simulink model "fixed_wing_sim"  (Simulink 8.7)
settings: Solver=ode4  StartTime=0.0  StopTime=T_sim  FixedStep=ts_sim  MaxStep=10e-3  RelTol=1e-3
InitFcn:
  | % Run the initialization script
  | clear all
  | aerosonde_uav_conf_model
StopFcn:
  | %show_result
  | print_results
values from neighbouring files (symbols this model uses):
  a = param(1)    [get_field.m]    (also in print_results.m = a*scale_fac/1e3; vector_field_parameters.m = 0.85)
  AilBnd = range_ail.*degrees2rad    [aerosonde_uav_conf_model.m]
  aileron_limits = [-20*pi/180;20*pi/180]    [aerosonde_uav_conf_model.m]
  AlphaBnd = range_alpha.*degrees2rad    [aerosonde_uav_conf_model.m]
  amp_theta = amp_theta*2    [vector_field_parameters.m]
  amp_theta_c = ((1/4)*[1 1 1]/6)*U_theta*tau_theta    [vector_field_parameters.m]
  amp_v_c = [1 1 1]*(tau_v*U_v)/6    [vector_field_parameters.m]
  amp_x = [5 5 5]    [vector_field_parameters.m]
  amp_y = [5 5 5]    [vector_field_parameters.m]
  amp_z = amp_z*2    [vector_field_parameters.m]
  amp_z_c = [1 1 1]*(tau_z*U_z)/6/2    [vector_field_parameters.m]
  b = param(2)    [get_field.m]    (also in print_results.m = b*scale_fac/1e3; vector_field_parameters.m = 0.08)
  BetaBnd = range_beta.*degrees2rad    [aerosonde_uav_conf_model.m]
  Bw = 2.8956    [aerosonde_uav_conf_model.m]
  c = param(3)    [get_field.m]    (also in vector_field_parameters.m = -0.13)
  CD_0 = 0.0434    [aerosonde_uav_conf_model.m]
  CD_ail = ones(length(AlphaBnd),1)*CD_aux_ail    [aerosonde_uav_conf_model.m]
  CD_alpha_beta = zeros(length(AlphaBnd),length(BetaBnd))    [aerosonde_uav_conf_model.m]
  CD_elev = ones(length(AlphaBnd),1)*CD_aux_elev    [aerosonde_uav_conf_model.m]
  CD_mind = 0.23    [aerosonde_uav_conf_model.m]
  CD_rud = ones(length(AlphaBnd),1)*CD_aux_rud    [aerosonde_uav_conf_model.m]
  CL_0 = 0.23    [aerosonde_uav_conf_model.m]
  Cl_ail = ones(length(AlphaBnd),1)*Cl_aux_ail    [aerosonde_uav_conf_model.m]
  CL_alpha_beta = CL_alpha*ones(1,length(BetaBnd))    [aerosonde_uav_conf_model.m]
  Cl_alpha_beta = ones(length(AlphaBnd),1)*Cl_beta    [aerosonde_uav_conf_model.m]
  CL_alphadot = 1.9724    [aerosonde_uav_conf_model.m]
  CL_elev = ones(length(AlphaBnd),1)*CL_aux_elev    [aerosonde_uav_conf_model.m]
  Cl_P = ones(length(AlphaBnd),1)*Cl_aux_P    [aerosonde_uav_conf_model.m]
  CL_Q = 7.9543*QBnd    [aerosonde_uav_conf_model.m]
  Cl_R = ones(length(AlphaBnd),1)*Cl_aux_R    [aerosonde_uav_conf_model.m]
  Cl_rud = ones(length(AlphaBnd),1)*Cl_aux_rud    [aerosonde_uav_conf_model.m]
  CLE_alphat = zeros(1,length(AlphaBnd))    [aerosonde_uav_conf_model.m]
  CLE_elev = 0    [aerosonde_uav_conf_model.m]
  Cm0 = 0.135    [aerosonde_uav_conf_model.m]
  Cm_alpha_beta = Cm_alpha*ones(1,length(BetaBnd))    [aerosonde_uav_conf_model.m]
  Cm_alphadot = -10.3796    [aerosonde_uav_conf_model.m]
  Cm_elev = ones(length(AlphaBnd),1)*Cm_aux_elev    [aerosonde_uav_conf_model.m]
  Cm_Q = -38.2067*QBnd    [aerosonde_uav_conf_model.m]
  Cn_ail = ones(length(AlphaBnd),1)*Cn_aux_ail    [aerosonde_uav_conf_model.m]
  Cn_alpha_beta = ones(length(AlphaBnd),1)*Cn_beta    [aerosonde_uav_conf_model.m]
  Cn_P = ones(length(AlphaBnd),1)*Cn_aux_P    [aerosonde_uav_conf_model.m]
  Cn_R = ones(length(AlphaBnd),1)*Cn_aux_R    [aerosonde_uav_conf_model.m]
  Cn_rud = ones(length(AlphaBnd),1)*Cn_aux_rud    [aerosonde_uav_conf_model.m]
  CT_save = CT_save.*10    [aerosonde_uav_conf_model.m]    (also in helice.mat = [0.115262 0.00375054783545 -0.00666475255621 -0.006665219028)
  curve = 1    [vector_field_parameters.m]
  Cw = 0.189941    [aerosonde_uav_conf_model.m]
  CY_ail = ones(length(AlphaBnd),1)*CY_aux_ail    [aerosonde_uav_conf_model.m]
  CY_alpha_beta = ones(length(AlphaBnd),1)*CY_beta    [aerosonde_uav_conf_model.m]
  CY_P = zeros(length(AlphaBnd),length(PBnd))    [aerosonde_uav_conf_model.m]
  CY_R = zeros(length(AlphaBnd),length(RBnd))    [aerosonde_uav_conf_model.m]
  CY_rud = ones(length(AlphaBnd),1)*CY_aux_rud    [aerosonde_uav_conf_model.m]
  d = param(4)    [get_field.m]    (also in vector_field_parameters.m = -0.04)
  D_hel = 0.15    [aerosonde_uav_conf_model.m]
  d_wash = 0    [aerosonde_uav_conf_model.m]
  delta_CD = 1    [aerosonde_uav_conf_model.m]
  delta_CL = 1    [aerosonde_uav_conf_model.m]
  delta_Cl = 1    [aerosonde_uav_conf_model.m]
  delta_Cm = 1    [aerosonde_uav_conf_model.m]
  delta_Cn = 1    [aerosonde_uav_conf_model.m]
  delta_CY = 1    [aerosonde_uav_conf_model.m]
  delta_FT = 1    [aerosonde_uav_conf_model.m]
  Delta_V_EH = [ 2 1.7365 1.2985 1.0890 1.0205]    [aerosonde_uav_conf_model.m]
  Delta_V_J = [ 0 0.4 0.7 1.4 2.1]    [aerosonde_uav_conf_model.m]
  elevator_limits = [-15*pi/180;15*pi/180]    [aerosonde_uav_conf_model.m]
  ElevBnd = range_elev.*degrees2rad    [aerosonde_uav_conf_model.m]
  F_T = 19    [aerosonde_uav_conf_model.m]
  f_theta = ([5 3 1]+rand(1,3))*0.05*2*pi/freq_divisor    [vector_field_parameters.m]
  f_theta_c = ([5 3 1]+rand(1,3))*0.05*2*pi/freq_divisor    [vector_field_parameters.m]
  f_v_c = ([4 2 0.5]+rand(1,3))*0.05*2*pi/freq_divisor    [vector_field_parameters.m]
  f_x = ([6 4 2]+rand(1,3))*0.05*2*pi/freq_divisor    [vector_field_parameters.m]
  f_y = ([6 4 2]+rand(1,3))*0.05*2*pi/freq_divisor    [vector_field_parameters.m]
  f_z = ([6 4 2]+rand(1,3))*0.05*2*pi/freq_divisor    [vector_field_parameters.m]
  f_z_c = ([4 2 0.5]+rand(1,3))*0.05*2*pi/freq_divisor    [vector_field_parameters.m]
  g1 = param(5)    [get_field.m]    (also in vector_field_parameters.m = 4)
  gain_G = param(6)    [get_field.m]    (also in vector_field_parameters.m = 2.5)
  gravity = 9.807    [aerosonde_uav_conf_model.m]
  H_0 = 200    [vector_field_parameters.m]
  Heq = 200    [aerosonde_uav_conf_model.m]    (also in vector_field_parameters.m)
  induced_drag = 1/(pi*AR*osw)    (= 0.0278403324809)    [aerosonde_uav_conf_model.m]
  isTrimming = 0    [aerosonde_uav_conf_model.m]
  J_save = J_save.*1.5    [aerosonde_uav_conf_model.m]    (also in helice.mat = [0 1.22229381539 1.27367709689 1.27367940534 1.27361400442 1)
  Jx = 0.7795    [aerosonde_uav_conf_model.m]
  Jxz = 0.1211    [aerosonde_uav_conf_model.m]
  Jy = 1.122    [aerosonde_uav_conf_model.m]
  Jz = 1.752    [aerosonde_uav_conf_model.m]
  KC_h = 0.28    [aerosonde_uav_conf_model.m]
  KC_phi = -1.18    [aerosonde_uav_conf_model.m]
  KC_psi = 0.03    [aerosonde_uav_conf_model.m]
  KC_r = -0.0073    [aerosonde_uav_conf_model.m]
  KC_theta = -1.1482    [aerosonde_uav_conf_model.m]
  KC_vt = 0.9948*1    (= 0.9948)    [aerosonde_uav_conf_model.m]
  KE = -0.1562    [aerosonde_uav_conf_model.m]
  Kp = 0.18    [vector_field_parameters.m]
  KR = 0.0130    (= 0.013)    [aerosonde_uav_conf_model.m]
  Ksad = param(3)    [get_field.m]    (also in print_results.m = Ksad*scale_fac/1e3; vector_field_parameters.m = 0)
  KT = 0.0792    [aerosonde_uav_conf_model.m]
  Kv = 1    [vector_field_parameters.m]
  LIM_CENTER = LIM_CENTER*scale_fac/1e3    [print_results.m]    (also in vector_field_parameters.m = 0.2)
  M = 8.5    [aerosonde_uav_conf_model.m]    (also in print_results.m = 0)
  motor_min = 0.1    [aerosonde_uav_conf_model.m]
  motor_rate = 1    [aerosonde_uav_conf_model.m]
  p_theta = rand(1,3)*2*pi    [vector_field_parameters.m]
  p_theta_c = rand(1,3)*2*pi    [vector_field_parameters.m]
  p_v_c = rand(1,3)*2*pi    [vector_field_parameters.m]
  p_x = rand(1,3)*2*pi    [vector_field_parameters.m]
  p_y = rand(1,3)*2*pi    [vector_field_parameters.m]
  p_z = rand(1,3)*2*pi    [vector_field_parameters.m]
  p_z_c = rand(1,3)*2*pi    [vector_field_parameters.m]
  PBnd = range_P.*degrees2rad    [aerosonde_uav_conf_model.m]
  perc_int_max = 0.8    [aerosonde_uav_conf_model.m]
  phi_max = 20*pi/180    (= 0.349065850399)    [aerosonde_uav_conf_model.m]
  phi_min = -20*pi/180    (= -0.349065850399)    [aerosonde_uav_conf_model.m]
  QBnd = range_Q.*degrees2rad    [aerosonde_uav_conf_model.m]
  r = sqrt(m)    [animation.m]    (also in print_results.m)
  r_aero_abc = r_aero_struct*[-1 0 0;0 1 0;0 0 -1]    [aerosonde_uav_conf_model.m]
  r_cg_abc = r_cg_struct*[-1 0 0;0 1 0;0 0 -1]    [aerosonde_uav_conf_model.m]
  r_motor_abc = r_motor_struct*[-1 0 0;0 1 0;0 0 -1]    [aerosonde_uav_conf_model.m]
  r_tail_abc = r_aero_struct*[-1 0 0;0 1 0;0 0 -1]    [aerosonde_uav_conf_model.m]
  RBnd = range_R.*degrees2rad    [aerosonde_uav_conf_model.m]
  rho = 0.1    [aerosonde_uav_conf_model.m]
  ... (+40 more)
undefined symbols (not defined in the file or in its folder): Earth, F, Light, MIL, WGS84
libraries: aerolibwind2 x2, aerolibtransform2 x2, aerolibfltsims x1, aerolibconvert2 x1, dspsigops x1
(part 3 of 3)

== system fixed_wing_sim/A/C + Low Level Control /UAV Internal Closed Loops/UAV model/Body-Axes 6DOF Equations/Moment Equations/Inverse Inertia Matrix ==
  Constant : Constant  Value=Jz
  Constant1 : Constant  Value=1/Jy
  Constant2 : Constant  Value=Jx
  Constant3 : Constant  Value=Jxz
  Constant4 : Constant  Value=0
  Constant5 : Constant  Value=Jx*Jz - Jxz^2
  Matrix Concatenation10 : Concatenate  NumInputs=3  Mode=Multidimensional array
  Matrix Concatenation11 : Concatenate  NumInputs=3  Mode=Multidimensional array  ConcatenateDimension=2
  Matrix Concatenation8 : Concatenate  NumInputs=3  Mode=Multidimensional array
  Matrix Concatenation9 : Concatenate  NumInputs=3  Mode=Multidimensional array
  Product : Product  Inputs=*/  SaturateOnIntegerOverflow=on  OutDataTypeStr=Inherit: Same as first input
  Product1 : Product  SaturateOnIntegerOverflow=on  OutDataTypeStr=Inherit: Same as first input
  inv J_b : Outport
  wires:
  Matrix Concatenation8/1 -> Matrix Concatenation11/1
  Matrix Concatenation9/1 -> Matrix Concatenation11/2
  Matrix Concatenation10/1 -> Matrix Concatenation11/3
  Constant/1 -> Matrix Concatenation8/1
  Constant4/1 -> Matrix Concatenation8/2, Matrix Concatenation9/1, Matrix Concatenation9/3, Matrix Concatenation10/2
  Constant3/1 -> Matrix Concatenation8/3, Matrix Concatenation10/1
  Constant2/1 -> Matrix Concatenation10/3
  Matrix Concatenation11/1 -> Product/1
  Product/1 -> inv J_b/1
  Constant5/1 -> Product/2, Product1/2
  Constant1/1 -> Product1/1
  Product1/1 -> Matrix Concatenation9/2

== system fixed_wing_sim/A/C + Low Level Control /UAV Internal Closed Loops/UAV model/Body-Axes 6DOF Equations/Moment Equations/Produto Vetorial1 ==
  V1 : Inport
  V2 : Inport  Port=2
  Mux : Mux  Inputs=2
  Mux1 : Mux  Inputs=3
  i : Fcn  Expr=u(2)*u(6)-u(3)*u(5)
  j : Fcn  Expr=-u(1)*u(6)+u(3)*u(4)
  k : Fcn  Expr=u(1)*u(5)-u(2)*u(4)
  V1 x V2 : Outport
  wires:
  V1/1 -> Mux/1
  V2/1 -> Mux/2
  Mux/1 -> i/1, j/1, k/1
  i/1 -> Mux1/1
  j/1 -> Mux1/2
  k/1 -> Mux1/3
  Mux1/1 -> V1 x V2/1

== system fixed_wing_sim/A/C + Low Level Control /UAV Internal Closed Loops/UAV model/Body-Axes 6DOF Equations/Moment Equations/Produto Vetorial2 ==
  V1 : Inport
  V2 : Inport  Port=2
  Mux : Mux  Inputs=2
  Mux1 : Mux  Inputs=3
  i : Fcn  Expr=u(2)*u(6)-u(3)*u(5)
  j : Fcn  Expr=-u(1)*u(6)+u(3)*u(4)
  k : Fcn  Expr=u(1)*u(5)-u(2)*u(4)
  V1 x V2 : Outport
  wires:
  V1/1 -> Mux/1
  V2/1 -> Mux/2
  Mux/1 -> i/1, j/1, k/1
  i/1 -> Mux1/1
  j/1 -> Mux1/2
  k/1 -> Mux1/3
  Mux1/1 -> V1 x V2/1

== system fixed_wing_sim/A/C + Low Level Control /UAV Internal Closed Loops/UAV model/Body-Axes 6DOF Equations/Moment Equations/Produto Vetorial3 ==
  V1 : Inport
  V2 : Inport  Port=2
  Mux : Mux  Inputs=2
  Mux1 : Mux  Inputs=3
  i : Fcn  Expr=u(2)*u(6)-u(3)*u(5)
  j : Fcn  Expr=-u(1)*u(6)+u(3)*u(4)
  k : Fcn  Expr=u(1)*u(5)-u(2)*u(4)
  V1 x V2 : Outport
  wires:
  V1/1 -> Mux/1
  V2/1 -> Mux/2
  Mux/1 -> i/1, j/1, k/1
  i/1 -> Mux1/1
  j/1 -> Mux1/2
  k/1 -> Mux1/3
  Mux1/1 -> V1 x V2/1

== system fixed_wing_sim/A/C + Low Level Control /UAV Internal Closed Loops/UAV model/Body-Axes 6DOF Equations/Moment Equations/Produto Vetorial4 ==
  V1 : Inport
  V2 : Inport  Port=2
  Mux : Mux  Inputs=2
  Mux1 : Mux  Inputs=3
  i : Fcn  Expr=u(2)*u(6)-u(3)*u(5)
  j : Fcn  Expr=-u(1)*u(6)+u(3)*u(4)
  k : Fcn  Expr=u(1)*u(5)-u(2)*u(4)
  V1 x V2 : Outport
  wires:
  V1/1 -> Mux/1
  V2/1 -> Mux/2
  Mux/1 -> i/1, j/1, k/1
  i/1 -> Mux1/1
  j/1 -> Mux1/2
  k/1 -> Mux1/3
  Mux1/1 -> V1 x V2/1

== system fixed_wing_sim/A/C + Low Level Control /UAV Internal Closed Loops/UAV model/Body-Axes 6DOF Equations/NED --> ABC/R_phi  ==
  note: 1       0      0
      | 0   cos   sin
      | 0  -sen  cos
  note: R_phi -->
  In1 : Inport
  Constant : Constant
  Constant1 : Constant  Value=0
  Gain : Gain  Gain=-1
  Matrix Concatenate : Concatenate  NumInputs=3  Mode=Multidimensional array
  Matrix Concatenate1 : Concatenate  NumInputs=3  Mode=Multidimensional array
  Matrix Concatenate2 : Concatenate  NumInputs=3  Mode=Multidimensional array
  Matrix Concatenate3 : Concatenate  NumInputs=3  Mode=Multidimensional array  ConcatenateDimension=2
  cos(phi) : Trigonometry  Operator=cos
  sin(phi) : Trigonometry
  Out1 : Outport
  wires:
  Constant/1 -> Matrix Concatenate/1
  Constant1/1 -> Matrix Concatenate/2, Matrix Concatenate/3, Matrix Concatenate1/1, Matrix Concatenate2/1
  cos(phi)/1 -> Matrix Concatenate1/2, Matrix Concatenate2/3
  sin(phi)/1 -> Gain/1, Matrix Concatenate2/2
  Gain/1 -> Matrix Concatenate1/3
  Matrix Concatenate/1 -> Matrix Concatenate3/1
  Matrix Concatenate1/1 -> Matrix Concatenate3/2
  Matrix Concatenate2/1 -> Matrix Concatenate3/3
  Matrix Concatenate3/1 -> Out1/1
  In1/1 -> cos(phi)/1, sin(phi)/1

== system fixed_wing_sim/A/C + Low Level Control /UAV Internal Closed Loops/UAV model/Body-Axes 6DOF Equations/NED --> ABC/R_psi ==
  note: cos  sin   0
      | -sin  cos  0
      | 0       0     1
  note: R_psi -->
  In1 : Inport
  Constant : Constant
  Constant1 : Constant  Value=0
  Gain : Gain  Gain=-1
  Matrix Concatenate : Concatenate  NumInputs=3  Mode=Multidimensional array
  Matrix Concatenate1 : Concatenate  NumInputs=3  Mode=Multidimensional array
  Matrix Concatenate2 : Concatenate  NumInputs=3  Mode=Multidimensional array
  Matrix Concatenate3 : Concatenate  NumInputs=3  Mode=Multidimensional array  ConcatenateDimension=2
  cos(phi) : Trigonometry  Operator=cos
  sin(phi) : Trigonometry
  Out1 : Outport
  wires:
  Matrix Concatenate/1 -> Matrix Concatenate3/1
  Matrix Concatenate1/1 -> Matrix Concatenate3/2
  Matrix Concatenate2/1 -> Matrix Concatenate3/3
  Matrix Concatenate3/1 -> Out1/1
  cos(phi)/1 -> Matrix Concatenate/1, Matrix Concatenate1/2
  Gain/1 -> Matrix Concatenate/2
  sin(phi)/1 -> Gain/1, Matrix Concatenate1/1
  Constant1/1 -> Matrix Concatenate/3, Matrix Concatenate1/3, Matrix Concatenate2/1, Matrix Concatenate2/2
  Constant/1 -> Matrix Concatenate2/3
  In1/1 -> cos(phi)/1, sin(phi)/1

== system fixed_wing_sim/A/C + Low Level Control /UAV Internal Closed Loops/UAV model/Body-Axes 6DOF Equations/NED --> ABC/R_theta ==
  note: cos  0 -sin
      | 0    1    0
      | sin   0  cos
  note: R_theta -->
  In1 : Inport
  Constant : Constant
  Constant1 : Constant  Value=0
  Gain : Gain  Gain=-1
  Matrix Concatenate : Concatenate  NumInputs=3  Mode=Multidimensional array
  Matrix Concatenate1 : Concatenate  NumInputs=3  Mode=Multidimensional array
  Matrix Concatenate2 : Concatenate  NumInputs=3  Mode=Multidimensional array
  Matrix Concatenate3 : Concatenate  NumInputs=3  Mode=Multidimensional array  ConcatenateDimension=2
  cos(phi) : Trigonometry  Operator=cos
  sin(phi) : Trigonometry
  Out1 : Outport
  wires:
  Matrix Concatenate/1 -> Matrix Concatenate3/1
  Matrix Concatenate1/1 -> Matrix Concatenate3/2
  Matrix Concatenate2/1 -> Matrix Concatenate3/3
  Matrix Concatenate3/1 -> Out1/1
  cos(phi)/1 -> Matrix Concatenate/1, Matrix Concatenate2/3
  Constant1/1 -> Matrix Concatenate/2, Matrix Concatenate1/1, Matrix Concatenate1/3, Matrix Concatenate2/2
  Constant/1 -> Matrix Concatenate1/2
  In1/1 -> cos(phi)/1, sin(phi)/1
  sin(phi)/1 -> Matrix Concatenate/3, Gain/1
  Gain/1 -> Matrix Concatenate2/1

== system fixed_wing_sim/A/C + Low Level Control /UAV Internal Closed Loops/UAV model/Body-Axes 6DOF Equations/Navigation Equations/ABC --> NED ==
  note: NED = (R_phi * R_theta * R_psi)^(T) * ABC
  attitude : Inport
  v_ABC : Inport  Port=2
  Bus Selector : BusSelector  OutputSignals=phi,theta,psi
  Math Function : Math  Operator=transpose  SaturateOnIntegerOverflow=on
  Product : Product  Multiplication=Matrix(*)  RndMeth=Zero
  Product1 : Product  Multiplication=Matrix(*)  RndMeth=Zero
  Product2 : Product  Multiplication=Matrix(*)  RndMeth=Zero
  "R_phi " : Subsystem
  R_psi : Subsystem
  R_theta : Subsystem
  NED : Outport
  wires:
  attitude/1 -> Bus Selector/1
  R_theta/1(Out1) -> Product/2
  Product/1 -> Product1/1
  "R_phi "/1(Out1) -> Product/1
  R_psi/1(Out1) -> Product1/2
  v_ABC/1 -> Product2/2
  Product2/1 -> NED/1
  Product1/1 -> Math Function/1
  Math Function/1 -> Product2/1
  Bus Selector/2 -> R_theta/1(In1)  "<theta>"
  Bus Selector/3 -> R_psi/1(In1)  "<psi>"
  Bus Selector/1 -> "R_phi "/1(In1)  "<phi>"

== system fixed_wing_sim/A/C + Low Level Control /UAV Internal Closed Loops/UAV model/Body-Axes 6DOF Equations/Force Equations/NED --> ABC/R_phi  ==
  note: 1       0      0
      | 0   cos   sin
      | 0  -sen  cos
  note: R_phi -->
  In1 : Inport
  Constant : Constant
  Constant1 : Constant  Value=0
  Gain : Gain  Gain=-1
  Matrix Concatenate : Concatenate  NumInputs=3  Mode=Multidimensional array
  Matrix Concatenate1 : Concatenate  NumInputs=3  Mode=Multidimensional array
  Matrix Concatenate2 : Concatenate  NumInputs=3  Mode=Multidimensional array
  Matrix Concatenate3 : Concatenate  NumInputs=3  Mode=Multidimensional array  ConcatenateDimension=2
  cos(phi) : Trigonometry  Operator=cos
  sin(phi) : Trigonometry
  Out1 : Outport
  wires:
  Constant/1 -> Matrix Concatenate/1
  Constant1/1 -> Matrix Concatenate/2, Matrix Concatenate/3, Matrix Concatenate1/1, Matrix Concatenate2/1
  cos(phi)/1 -> Matrix Concatenate1/2, Matrix Concatenate2/3
  sin(phi)/1 -> Gain/1, Matrix Concatenate2/2
  Gain/1 -> Matrix Concatenate1/3
  Matrix Concatenate/1 -> Matrix Concatenate3/1
  Matrix Concatenate1/1 -> Matrix Concatenate3/2
  Matrix Concatenate2/1 -> Matrix Concatenate3/3
  Matrix Concatenate3/1 -> Out1/1
  In1/1 -> cos(phi)/1, sin(phi)/1

== system fixed_wing_sim/A/C + Low Level Control /UAV Internal Closed Loops/UAV model/Body-Axes 6DOF Equations/Force Equations/NED --> ABC/R_psi ==
  note: cos  sin   0
      | -sin  cos  0
      | 0       0     1
  note: R_psi -->
  In1 : Inport
  Constant : Constant
  Constant1 : Constant  Value=0
  Gain : Gain  Gain=-1
  Matrix Concatenate : Concatenate  NumInputs=3  Mode=Multidimensional array
  Matrix Concatenate1 : Concatenate  NumInputs=3  Mode=Multidimensional array
  Matrix Concatenate2 : Concatenate  NumInputs=3  Mode=Multidimensional array
  Matrix Concatenate3 : Concatenate  NumInputs=3  Mode=Multidimensional array  ConcatenateDimension=2
  cos(phi) : Trigonometry  Operator=cos
  sin(phi) : Trigonometry
  Out1 : Outport
  wires:
  Matrix Concatenate/1 -> Matrix Concatenate3/1
  Matrix Concatenate1/1 -> Matrix Concatenate3/2
  Matrix Concatenate2/1 -> Matrix Concatenate3/3
  Matrix Concatenate3/1 -> Out1/1
  cos(phi)/1 -> Matrix Concatenate/1, Matrix Concatenate1/2
  Gain/1 -> Matrix Concatenate/2
  sin(phi)/1 -> Gain/1, Matrix Concatenate1/1
  Constant1/1 -> Matrix Concatenate/3, Matrix Concatenate1/3, Matrix Concatenate2/1, Matrix Concatenate2/2
  Constant/1 -> Matrix Concatenate2/3
  In1/1 -> cos(phi)/1, sin(phi)/1

== system fixed_wing_sim/A/C + Low Level Control /UAV Internal Closed Loops/UAV model/Body-Axes 6DOF Equations/Force Equations/NED --> ABC/R_theta ==
  note: cos  0 -sin
      | 0    1    0
      | sin   0  cos
  note: R_theta -->
  In1 : Inport
  Constant : Constant
  Constant1 : Constant  Value=0
  Gain : Gain  Gain=-1
  Matrix Concatenate : Concatenate  NumInputs=3  Mode=Multidimensional array
  Matrix Concatenate1 : Concatenate  NumInputs=3  Mode=Multidimensional array
  Matrix Concatenate2 : Concatenate  NumInputs=3  Mode=Multidimensional array
  Matrix Concatenate3 : Concatenate  NumInputs=3  Mode=Multidimensional array  ConcatenateDimension=2
  cos(phi) : Trigonometry  Operator=cos
  sin(phi) : Trigonometry
  Out1 : Outport
  wires:
  Matrix Concatenate/1 -> Matrix Concatenate3/1
  Matrix Concatenate1/1 -> Matrix Concatenate3/2
  Matrix Concatenate2/1 -> Matrix Concatenate3/3
  Matrix Concatenate3/1 -> Out1/1
  cos(phi)/1 -> Matrix Concatenate/1, Matrix Concatenate2/3
  Constant1/1 -> Matrix Concatenate/2, Matrix Concatenate1/1, Matrix Concatenate1/3, Matrix Concatenate2/2
  Constant/1 -> Matrix Concatenate1/2
  In1/1 -> cos(phi)/1, sin(phi)/1
  sin(phi)/1 -> Matrix Concatenate/3, Gain/1
  Gain/1 -> Matrix Concatenate2/1

== system fixed_wing_sim/A/C + Low Level Control /UAV Internal Closed Loops/UAV model/Body-Axes 6DOF Equations/Navigation Equations/ABC --> NED/R_phi  ==
  note: 1       0      0
      | 0   cos   sin
      | 0  -sen  cos
  note: R_phi -->
  In1 : Inport
  Constant : Constant
  Constant1 : Constant  Value=0
  Gain : Gain  Gain=-1
  Matrix Concatenate : Concatenate  NumInputs=3  Mode=Multidimensional array
  Matrix Concatenate1 : Concatenate  NumInputs=3  Mode=Multidimensional array
  Matrix Concatenate2 : Concatenate  NumInputs=3  Mode=Multidimensional array
  Matrix Concatenate3 : Concatenate  NumInputs=3  Mode=Multidimensional array  ConcatenateDimension=2
  cos(phi) : Trigonometry  Operator=cos
  sin(phi) : Trigonometry
  Out1 : Outport
  wires:
  Constant/1 -> Matrix Concatenate/1
  Constant1/1 -> Matrix Concatenate/2, Matrix Concatenate/3, Matrix Concatenate1/1, Matrix Concatenate2/1
  cos(phi)/1 -> Matrix Concatenate1/2, Matrix Concatenate2/3
  sin(phi)/1 -> Gain/1, Matrix Concatenate2/2
  Gain/1 -> Matrix Concatenate1/3
  Matrix Concatenate/1 -> Matrix Concatenate3/1
  Matrix Concatenate1/1 -> Matrix Concatenate3/2
  Matrix Concatenate2/1 -> Matrix Concatenate3/3
  Matrix Concatenate3/1 -> Out1/1
  In1/1 -> cos(phi)/1, sin(phi)/1

== system fixed_wing_sim/A/C + Low Level Control /UAV Internal Closed Loops/UAV model/Body-Axes 6DOF Equations/Navigation Equations/ABC --> NED/R_psi ==
  note: cos  sin   0
      | -sin  cos  0
      | 0       0     1
  note: R_psi -->
  In1 : Inport
  Constant : Constant
  Constant1 : Constant  Value=0
  Gain : Gain  Gain=-1
  Matrix Concatenate : Concatenate  NumInputs=3  Mode=Multidimensional array
  Matrix Concatenate1 : Concatenate  NumInputs=3  Mode=Multidimensional array
  Matrix Concatenate2 : Concatenate  NumInputs=3  Mode=Multidimensional array
  Matrix Concatenate3 : Concatenate  NumInputs=3  Mode=Multidimensional array  ConcatenateDimension=2
  cos(phi) : Trigonometry  Operator=cos
  sin(phi) : Trigonometry
  Out1 : Outport
  wires:
  Matrix Concatenate/1 -> Matrix Concatenate3/1
  Matrix Concatenate1/1 -> Matrix Concatenate3/2
  Matrix Concatenate2/1 -> Matrix Concatenate3/3
  Matrix Concatenate3/1 -> Out1/1
  cos(phi)/1 -> Matrix Concatenate/1, Matrix Concatenate1/2
  Gain/1 -> Matrix Concatenate/2
  sin(phi)/1 -> Gain/1, Matrix Concatenate1/1
  Constant1/1 -> Matrix Concatenate/3, Matrix Concatenate1/3, Matrix Concatenate2/1, Matrix Concatenate2/2
  Constant/1 -> Matrix Concatenate2/3
  In1/1 -> cos(phi)/1, sin(phi)/1

== system fixed_wing_sim/A/C + Low Level Control /UAV Internal Closed Loops/UAV model/Body-Axes 6DOF Equations/Navigation Equations/ABC --> NED/R_theta ==
  note: cos  0 -sin
      | 0    1    0
      | sin   0  cos
  note: R_theta -->
  In1 : Inport
  Constant : Constant
  Constant1 : Constant  Value=0
  Gain : Gain  Gain=-1
  Matrix Concatenate : Concatenate  NumInputs=3  Mode=Multidimensional array
  Matrix Concatenate1 : Concatenate  NumInputs=3  Mode=Multidimensional array
  Matrix Concatenate2 : Concatenate  NumInputs=3  Mode=Multidimensional array
  Matrix Concatenate3 : Concatenate  NumInputs=3  Mode=Multidimensional array  ConcatenateDimension=2
  cos(phi) : Trigonometry  Operator=cos
  sin(phi) : Trigonometry
  Out1 : Outport
  wires:
  Matrix Concatenate/1 -> Matrix Concatenate3/1
  Matrix Concatenate1/1 -> Matrix Concatenate3/2
  Matrix Concatenate2/1 -> Matrix Concatenate3/3
  Matrix Concatenate3/1 -> Out1/1
  cos(phi)/1 -> Matrix Concatenate/1, Matrix Concatenate2/3
  Constant1/1 -> Matrix Concatenate/2, Matrix Concatenate1/1, Matrix Concatenate1/3, Matrix Concatenate2/2
  Constant/1 -> Matrix Concatenate1/2
  In1/1 -> cos(phi)/1, sin(phi)/1
  sin(phi)/1 -> Matrix Concatenate/3, Gain/1
  Gain/1 -> Matrix Concatenate2/1

== matlab function Control Law/Control law ==
  data: theta_c output double; x input double; v_c output double; z_c output double; y input double; xd input double; yd input double; theta input double; z input double; zd input double; V_theta output double; V_fld output double; v_min parameter double; b parameter double; tau_theta parameter double; Kp parameter double; Kv parameter double; Veq parameter double; Heq parameter double; Ksad parameter double; c parameter double; LIM_CENTER parameter double; curve parameter double; tau_z parameter double; g1 parameter double; scale_fac parameter double; gain_G parameter double; vz_max parameter double; v_max parameter double; a parameter double; d parameter double; teste output double
function [theta_c, v_c, z_c, V_theta, V_fld, teste] = ControlLaw(x,y,xd,yd,theta,z,zd, v_min, b, tau_theta, Kp, Kv, Veq, Heq, Ksad, c, LIM_CENTER, curve, tau_z, g1, scale_fac, gain_G, vz_max, v_max, a, d)


v_ref = Veq; %~23

%Point in which the field will be evaluated
xn = x;
yn = y;
zn = z-Heq; %!!!!!!!!!!!!!!

%Scalling the vector field
xn = xn/scale_fac;
yn = yn/scale_fac;
zn = zn/scale_fac;

v = sqrt(xd^2 + yd^2);

%Field evaluatioin
if (curve == 1) % Saddle/Ellipse
    [Vxyz, conv_V, circ_V, Vxyz_hat, alpha_1, alpha_2, v_alpha] = get_field([xn,yn,zn],[a,b,Ksad,g1,gain_G],'saddle');
    Vx0 = Vxyz(1); Vy0 = Vxyz(2); Vz0 = Vxyz(3);
    
elseif (curve == 2) % Shape
    [Vxyz, conv_V, circ_V, Vxyz_hat, alpha_1, alpha_2, v_alpha] = get_field([xn,yn,zn],[a,b,c,g1,gain_G],'shape');
    Vx0 = Vxyz(1); Vy0 = Vxyz(2); Vz0 = Vxyz(3);
    
elseif (curve == 3) % Random
    [Vxyz, conv_V, circ_V, Vxyz_hat, alpha_1, alpha_2, v_alpha] = get_field([xn,yn,zn],[a,b,c,g1,gain_G],'random');
    Vx0 = Vxyz(1); Vy0 = Vxyz(2); Vz0 = Vxyz(3);
        
elseif (curve == 4) % Polynomial open curve
    [Vxyz, conv_V, circ_V, Vxyz_hat, alpha_1, alpha_2, v_alpha] = get_field([xn,yn,zn],[a,b,c,d,g1,gain_G],'poly');
    Vx0 = Vxyz(1); Vy0 = Vxyz(2); Vz0 = Vxyz(3);
    
else
    Vx0 = 0;
    Vy0 = 0;
    Vz0 = 0;
    v_alpha = 0;
end
%Vector normalization
absValue = (Vx0^2 + Vy0^2 + 0*Vz0^2)^0.5; %normalize only on (x,y)
Vx = Vx0/absValue;
Vy = Vy0/absValue;
Vz = Vz0/absValue;


%Compute the curl and the divergence
if (curve == 1) % Saddle/Ellipse
    [G_Phi_x,G_Phi_y] = get_grad([xn,yn,zn],[a,b,Ksad,g1,gain_G],'saddle');
%     [CURL,DIV] = get_curl_div([xn,yn,zn],[a,b,Ksad,g1,gain_G],'saddle');
elseif (curve == 2) % Shape
    [G_Phi_x,G_Phi_y] = get_grad([xn,yn,zn],[a,b,c,g1,gain_G],'shape');
%     [CURL,DIV] = get_curl_div([xn,yn,zn],[a,b,c,g1,gain_G],'shape');
elseif (curve == 3) % Random
    [G_Phi_x,G_Phi_y] = get_grad([xn,yn,zn],[a,b,c,g1,gain_G],'random');
%     [CURL,DIV] = get_curl_div([xn,yn,zn],[a,b,c,g1,gain_G],'random');
elseif (curve == 4) % Polynomial
    [G_Phi_x,G_Phi_y] = get_grad([xn,yn,zn],[a,b,c,d,g1,gain_G],'poly');
%     [CURL,DIV] = get_curl_div([xn,yn,zn],[a,b,c,d,g1,gain_G],'poly');
else
	G_Phi_x = 0;
    G_Phi_y = 0;
    CURL = 0;
    DIV = 0;
end


%Compute the orientation of the local field
theta_f = atan2(Vy,Vx);

% sin and cos of the orientation error
sin_erro_theta = sin(atan2(Vy,Vx)-theta);
cos_erro_theta = cos(atan2(Vy,Vx)-theta);

%Forward speed reference
v_c = v_ref;
% k1 = (v_c+v_min)/2; k2 = (v_c-v_min)/2;
% v_c = k1 + k2*cos_erro_theta;
v_c = v + Kv*(-v+v_c);

%Height controll
Vz_tilde = (v/absValue)*Vz0; % = v*Vz
Vz_c = Vz_tilde;
if(abs(Vz_c) > vz_max)
    Vz_c = (Vz_c/abs(Vz_c))*vz_max;
end
Vz_c = Vz_c;

w_c = Kp*sin_erro_theta + [Vx*G_Phi_y - Vy*G_Phi_x]'*[xd; yd; zd]/scale_fac;
% [Vx*G_Phi_y - Vy*G_Phi_x]'*[xd; yd; zd]/scale_fac
% w_c = Kp*sin_erro_theta + v*(cos(theta_f-theta)*CURL - sin(theta_f-theta)*DIV)/scale_fac;
% w_c = w_c - 0.06*-1;
% w_c = w_c - 0.04;


%If inside the circle around the singularity
if (curve ~= 4)
    if (norm([xn,yn]) < LIM_CENTER)
        w_c = 0;
        Vz_c = 0;
    end
end



v_c = v_c;

theta_c = tau_theta*w_c + theta;

z_c = tau_z*Vz_c + (zn*scale_fac+Heq);




% Orientation Lyaunov function
V_theta = 1-cos(theta-theta_f);

% Field Potential function
V_fld = v_alpha;


teste = [Vx, Vy, norm(G_Phi_x), norm(G_Phi_y), xd, yd, zd, [Vx*G_Phi_y - Vy*G_Phi_x]'*[xd; yd; zd]/scale_fac, Kp*sin_erro_theta];
